simulink model "sf_cpp"  (Simulink 6.0)
settings: Solver=FixedStepDiscrete  StartTime=0.0  StopTime=inf  RelTol=1e-3
libraries: simulink x1
settings Model: CovMetricSettings=dcmtr  Creator=The MathWorks Inc.  LastModifiedBy=batserve  ExtModeAutoUpdateStatusClock=off
settings DataIOCC: SignalLoggingName=sigsOut
settings OptimizationCC: InlineInvariantSignals=off
settings DebuggingCC: CheckExecutionContextPreStartOutputMsg=on  CheckExecutionContextRuntimeOutputMsg=on  SolverPrmCheckMsg=none
settings HardwareCC: TargetHWDeviceType=32-bit Generic  ProdEqTarget=off
settings RTWCC: CustomSourceCode="#include \"adder_cpp.h\""  CustomInclude=./custom_cpp_src  CustomSource=./custom_cpp_src/adder_cpp.cpp  CustomInitializer=adderVar = createAdder();  CustomTerminator=deleteAdder(adderVar);

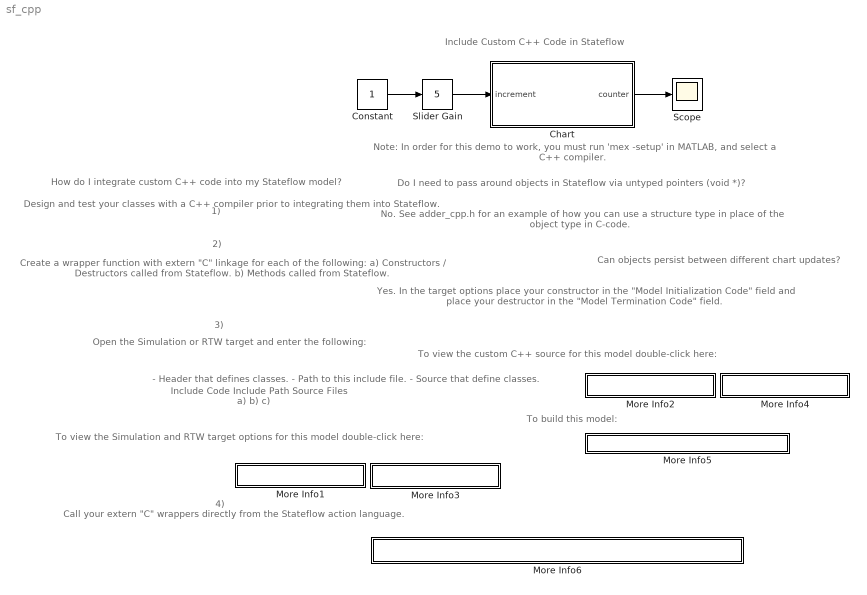
== system sf_cpp ==
  note: Include Custom C++ Code in Stateflow
  note: How do I integrate custom C++ code into my Stateflow
      | model?
  note: To view the Simulation and RTW target options
      | for this model double-click here:
  note: Can objects persist between different chart updates?
  note: Yes.  In the target options place your constructor in the
      | "Model Initialization Code" field and place your
      | destructor in the "Model Termination Code" field.
  note: Do I need to pass around objects in Stateflow via
      | untyped pointers (void *)?
  note: No.  See adder_cpp.h for an example of how you can
      | use a structure type in place of the object type in C-code.
  note: Open the Simulation or RTW target and enter the
      | following:
  note: 1)
  note: 4)
  note: Call your extern "C" wrappers directly from the Stateflow
      | action language.
  note: Design and test your classes with a C++
      | compiler prior to integrating them into Stateflow.
  note: Create a wrapper function with extern "C" linkage
      | for each of the following:
      |
      |    a) Constructors / Destructors called from Stateflow.
      |    b) Methods called from Stateflow.
  note: Include Code
      | Include Path
      | Source Files
  note: - Header that defines classes.
      | - Path to this include file.
      | - Source that define classes.
  note: a)
      | b)
      | c)
  note: 2)
  note: 3)
  note: To view the custom C++ source for this model
      | double-click here:
  note: Note: In order for this demo to work, you must run 'mex -setup' in MATLAB, and select a C++ compiler.
  note: To build this model:
  Chart : Stateflow chart  PropExecContextAcrossSSBoundary=on
  Constant : Constant
  More Info1 : Subsystem  PropExecContextAcrossSSBoundary=on
      settings: OpenFcn=|
      | rt=sfroot;
      | m=rt.find('-isa','Stateflow.Machine','-and', 'name','sf_cpp');
      | tar=m.find('-isa','Stateflow.Target','-and','name','sfun');
      | sf('Private','targetddg_btn_target_cb',tar,'Target Options');
      mask Display: disp('Simulation target')
  More Info2 : Subsystem  PropExecContextAcrossSSBoundary=on
      settings: OpenFcn=|
      | filename=fullfile(matlabroot, 'toolbox', 'stateflow', 'sfdemos', 'custom_cpp_src', 'adder_cpp.cpp');
      | eval('edit(filename)')
      mask Display: disp('adder_cpp.cpp')
  More Info3 : Subsystem  PropExecContextAcrossSSBoundary=on
      settings: OpenFcn=|
      | slCfgPrmDlg(bdroot,'Open');
      | slCfgPrmDlg(bdroot,'TurnToPage','Custom Code');
      mask Display: disp('RTW target')
  More Info4 : Subsystem  PropExecContextAcrossSSBoundary=on
      settings: OpenFcn=|
      | filename=fullfile(matlabroot, 'toolbox', 'stateflow', 'sfdemos', 'custom_cpp_src', 'adder_cpp.h');
      | eval('edit(filename)')
      mask Display: disp('adder_cpp.h')
  More Info5 : Subsystem  PropExecContextAcrossSSBoundary=on
      settings: OpenFcn=rtwbuild('sf_cpp')
      mask Display: disp('Double click to build model')
  More Info6 : Subsystem  PropExecContextAcrossSSBoundary=on
      settings: OpenFcn=|
      | filename=fullfile(matlabroot, 'toolbox', 'stateflow', 'sfdemos', 'custom_cpp_src', 'adder_cpp.cpp');
      | eval('edit(filename)')
      mask Display: disp('matlabroot\toolbox\stateflow\sfdemos\custom_cpp_src\adder_cpp.cpp')
  Scope : Scope
      settings: YMin=15  YMax=105
  Slider Gain : simulink/Math Operations/Slider Gain  low=0  gain=5  high=5
  wires:
  Constant/1 -> Slider Gain/1
  Slider Gain/1 -> Chart/1(increment)
  Chart/1(counter) -> Scope/1

== system sf_cpp/More Info1 ==

== system sf_cpp/More Info2 ==

== system sf_cpp/More Info3 ==

== system sf_cpp/More Info4 ==

== system sf_cpp/More Info5 ==

== system sf_cpp/More Info6 ==

== stateflow chart Chart ==
  state under_100
    during: counter = adderOutput(adderVar, increment);
  state over_100
    during: counter = adderOutput(adderVar, -increment);
  note: NOTE: Please see "Target Options" for calls to
      |            constructor and destructor.
  (default) -> under_100 : / counter = 0;
  under_100 -> over_100 : [counter > 100]
  over_100 -> under_100 : [counter < 0]
  data: increment input int32 size=1; counter output double size=1
